simulink model "Simulink_UI_Test"  (R2025b)
settings: Solver=FixedStepAuto  StartTime=0.0  StopTime=inf  RelTol=1e-3
settings Model: SimulationMode=external  Creator=kueh_js  LastModifiedBy=kueh_js
settings OptimizationCC: OptimizeBlockIOStorage=off  EnhancedBackFolding=on  PassReuseOutputArgsThreshold=0.0  ZeroExternalMemoryAtStartup=off  ZeroInternalMemoryAtStartup=off  OptimizeBlockOrder=speed  DifferentSizesBufferReuse=on
settings DebuggingCC: ParameterTunabilityLossMsg=error
settings HardwareCC: ProdBitPerLong=64.0  ProdHWDeviceType=Intel->x86-64 (Linux 64)
settings SFSimCC: MATLABDynamicMemAlloc=off  SimTargetLang=C++  SimDLTargetLibrary=mkl-dnn
settings RTWCC: GenCodeOnly=on  Toolchain=GNU gcc/g++ | gmake (64-bit Linux)  TargetLang=C++
settings CodeAppCC: ForceParamTrailComments=on  OperatorAnnotations=on  MATLABSourceComments=on
settings GRTTargetCC: TargetLangStandard=C++20 (ISO)  MatFileLogging=off  CodeInterfacePackaging=C++ class

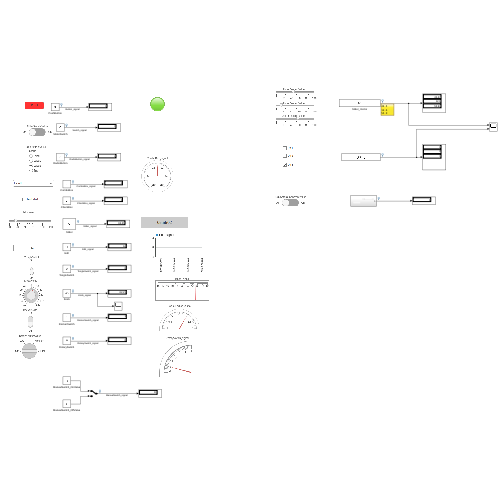
[thumbnail: Simulink's stored preview of the top-level diagram]
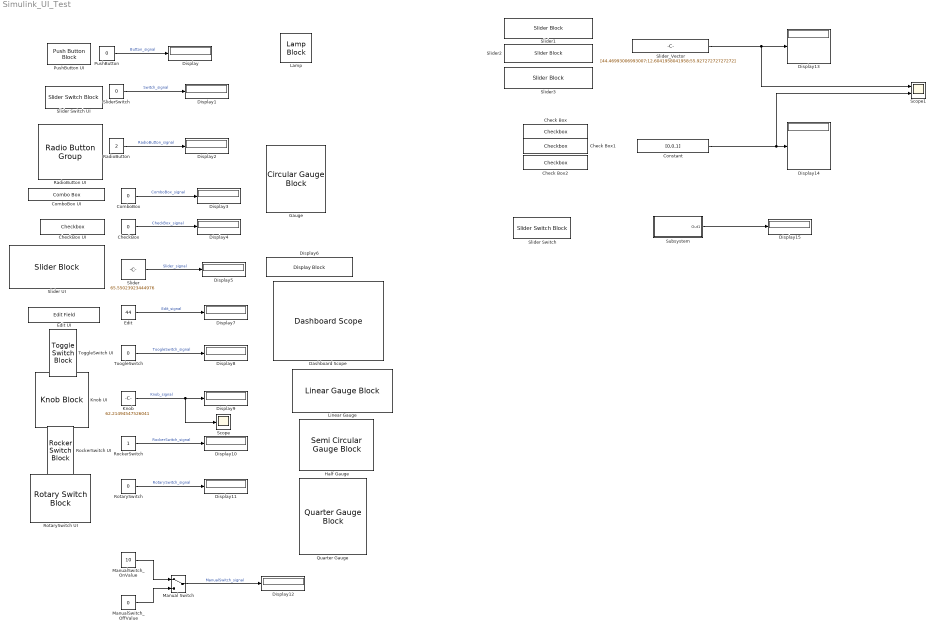
== system Simulink_UI_Test ==
  Check Box : Checkbox  LabelPosition=Hide  ShowInitialText=on  Label=On 1  Values=[0.0, 1.0]
  Check Box1 : Checkbox  LabelPosition=Hide  ShowInitialText=on  Label=On 2  Values=[0.0, 1.0]
  Check Box2 : Checkbox  LabelPosition=Hide  ShowInitialText=on  Label=On 3  Values=[0.0, 1.0]
  CheckBox : Constant  Value=0  OutDataTypeStr=boolean
  CheckBox UI : Checkbox  LabelPosition=Hide  ShowInitialText=on  Label=TestLabel  Values=[0.0, 1.0]
  ComboBox : Constant  Value=0  OutDataTypeStr=uint64
  ComboBox UI : ComboBox  LabelPosition=Hide
  Constant : Constant  Value=[0,0,1]
  Dashboard Scope : DashboardScope  FontColor=[0.0, 0.0, 0.0]
  Display{,1..5,7..15} (15 alike) : Display
  Display6 : DisplayBlock  LabelPosition=Hide  Transparency=1  GridColor=[0.502, 0.502, 0.502]
  Edit : Constant  Value=44  OutDataTypeStr=double
  Edit UI : EditField  LabelPosition=Hide  ShowInitialText=on  Alignment=Center
  Gauge : CircularGaugeBlock  ScaleMin=-110  ScaleMax=110  FontColor=[0.0, 0.0, 0.0]
  Half Gauge : SemiCircularGaugeBlock  ScaleMin=-1  ScaleMax=2  FontColor=[0.0, 0.0, 0.0]
  Knob : Constant  Value=62.21494547526041  OutDataTypeStr=double
  Knob UI : KnobBlock  ScaleMin=-10  ScaleMax=120
  Lamp : LampBlock  LabelPosition=Hide  DefaultColor=[192.0, 192.0, 192.0]
  Linear Gauge : LinearGaugeBlock  ScaleMin=10  ScaleMax=80  FontColor=[0.0, 0.0, 0.0]
  Manual Switch : ManualSwitch
  ManualSwitch_OffValue : Constant  Value=0
  ManualSwitch_OnValue : Constant  Value=10
  PushButton : Constant  Value=0  OutDataTypeStr=boolean
  PushButton UI : PushButtonBlock  ButtonText=Reset  IconOnColor=[0.0, 0.39215686274509803, 0.0]  IconOffColor=[0.0, 1.0, 0.0]  OffValue=0.000000
  Quarter Gauge : QuarterGaugeBlock  ScaleMin=-1  ScaleMax=5  FontColor=[0.0, 0.0, 0.0]
  RadioButton : Constant  Value=2  OutDataTypeStr=uint64
  RadioButton UI : RadioButtonGroup  SelectedLabel=Label3  ButtonGroupName=Group
  RockerSwitch : Constant  OutDataTypeStr=boolean
  RockerSwitch UI : RockerSwitchBlock
  RotarySwitch : Constant  Value=0  OutDataTypeStr=int64
  RotarySwitch UI : RotarySwitchBlock
  Scope : Scope
  Scope1 : Scope  NumInputPorts=2
  Slider : Constant  Value=65.55023923444976  OutDataTypeStr=double
  Slider Switch : SliderSwitchBlock
  Slider Switch UI : SliderSwitchBlock
  Slider UI : SliderBlock  ScaleMin=50  ScaleMax=150
  Slider1 : SliderBlock
  Slider2 : SliderBlock
  Slider3 : SliderBlock
  SliderSwitch : Constant  Value=0  OutDataTypeStr=boolean
  Slider_Vector : Constant  Value=[44.46993006993007;12.6041958041958;55.92727272727272]
  Subsystem : Subsystem
  ToggleSwitch UI : ToggleSwitchBlock
  ToogleSwitch : Constant  Value=0  OutDataTypeStr=boolean
  wires:
  Slider/1 -> Display5/1  "Slider_signal"
  ComboBox/1 -> Display3/1  "ComboBox_signal"
  CheckBox/1 -> Display4/1  "CheckBox_signal"
  PushButton/1 -> Display/1  "Button_signal"
  RadioButton/1 -> Display2/1  "RadioButton_signal"
  SliderSwitch/1 -> Display1/1  "Switch_signal"
  Edit/1 -> Display7/1  "Edit_signal"
  ToogleSwitch/1 -> Display8/1  "ToogleSwitch_signal"
  Knob/1 -> Scope/1, Display9/1  "Knob_signal"
  RockerSwitch/1 -> Display10/1  "RockerSwitch_signal"
  RotarySwitch/1 -> Display11/1  "RotarySwitch_signal"
  Manual Switch/1 -> Display12/1  "ManualSwitch_signal"
  ManualSwitch_OnValue/1 -> Manual Switch/1
  ManualSwitch_OffValue/1 -> Manual Switch/2
  Slider_Vector/1 -> Display13/1, Scope1/1
  Constant/1 -> Display14/1, Scope1/2
  Subsystem/1(Out1) -> Display15/1

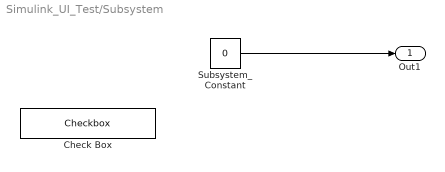
== system Simulink_UI_Test/Subsystem ==
  Check Box : Checkbox  LabelPosition=Hide  ShowInitialText=on  Values=[0.0, 1.0]
  Subsystem_Constant : Constant  Value=0
  Out1 : Outport
  wires:
  Subsystem_Constant/1 -> Out1/1
